simulink model "Control"  (R2024b)
settings: Solver=VariableStepAuto  StartTime=0.0  StopTime=10.0  RelTol=1e-3
values from neighbouring files (symbols this model uses):
  B = [0; 1/m]    [PaT.m]    (also in VanDerPol.m = [0; 1]; phase_portrait_pendulum.m = [0; 1/m*l])
  g = 9.81    [phase_portrait_pendulum.m]
undefined symbols (not defined in the file or in its folder): K, K1, Ke, Kt, L, Lm, m0, m1, N, R, r
settings Model: Creator=Anfisa Konycheva  LastModifiedBy=Anfisa Konycheva

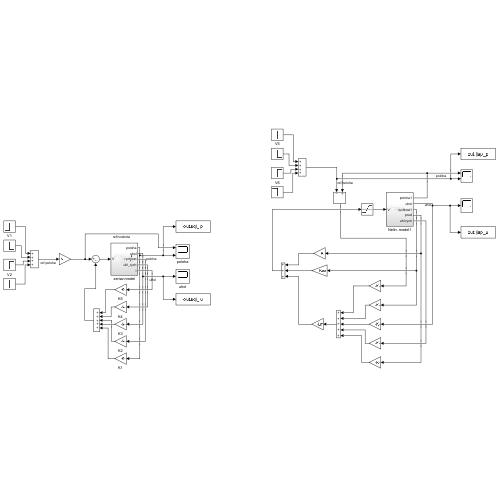
[thumbnail: Simulink's stored preview of the top-level diagram]
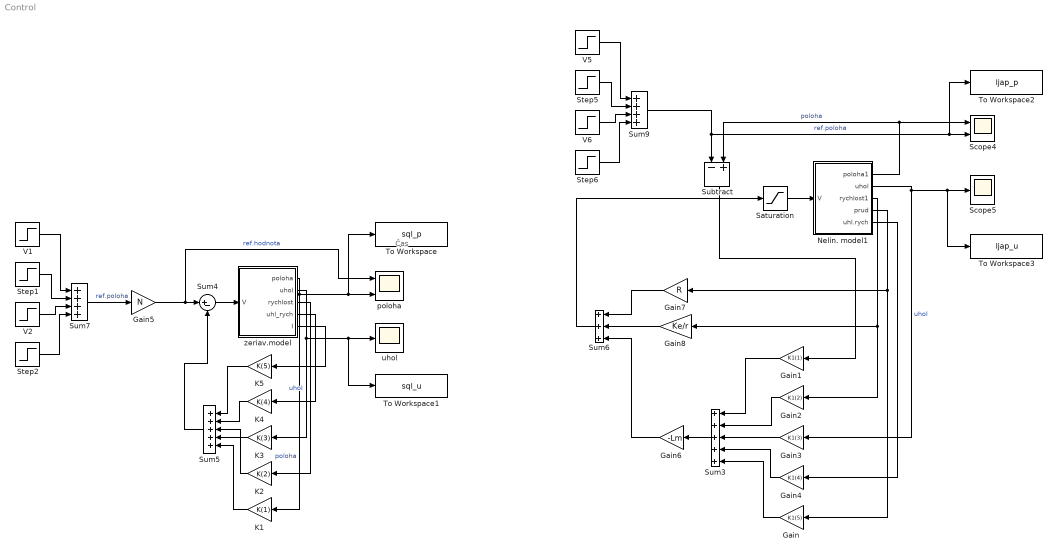
== system Control ==
  note: Čas
  Gain : Gain  Gain=K1(5)
  Gain1 : Gain  Gain=K1(1)
  Gain2 : Gain  Gain=K1(2)
  Gain3 : Gain  Gain=K1(3)
  Gain4 : Gain  Gain=K1(4)
  Gain5 : Gain  Gain=N
  Gain6 : Gain  Gain=-Lm
  Gain7 : Gain  Gain=R
  Gain8 : Gain  Gain=Ke/r
  K1 : Gain  Gain=K(1)
  K2 : Gain  Gain=K(2)
  K3 : Gain  Gain=K(3)
  K4 : Gain  Gain=K(4)
  K5 : Gain  Gain=K(5)
  Nelin. model1 : Subsystem
  Saturation : Saturate  UpperLimit=10  LowerLimit=-10
  Scope4 : Scope  NumInputPorts=2
  Scope5 : Scope
  Step1 : Step  Time=40  After=-5  SampleTime=0
  Step2 : Step  Time=80  After=-5  SampleTime=0
  Step5 : Step  Time=40  After=-5  SampleTime=0
  Step6 : Step  Time=80  After=-5  SampleTime=0
  Subtract : Sum  Inputs=-+
  Sum3 : Sum  Inputs=+++++
  Sum4 : Sum  Inputs=|+-
  Sum5 : Sum  Inputs=+++++
  Sum6 : Sum  Inputs=+++
  Sum7 : Sum  Inputs=++++
  Sum9 : Sum  Inputs=++++
  To Workspace : ToWorkspace  VariableName=sql_p  SaveFormat=Timeseries  SampleTime=-1
  To Workspace1 : ToWorkspace  VariableName=sql_u  SaveFormat=Timeseries  SampleTime=-1
  To Workspace2 : ToWorkspace  VariableName=ljap_p  SaveFormat=Timeseries  SampleTime=-1
  To Workspace3 : ToWorkspace  VariableName=ljap_u  SaveFormat=Timeseries  SampleTime=-1
  V1 : Step  Time=10  After=5  SampleTime=0
  V2 : Step  Time=60  After=5  SampleTime=0
  V5 : Step  Time=10  After=5  SampleTime=0
  V6 : Step  Time=60  After=5  SampleTime=0
  poloha : Scope  NumInputPorts=2
  uhol : Scope
  zeriav.model : Subsystem
  wires:
  K1/1 -> Sum5/5
  zeriav.model/1(poloha) -> K1/1, To Workspace/1, poloha/2  "poloha"
  V5/1 -> Sum9/1
  V6/1 -> Sum9/3
  Saturation/1 -> Nelin. model1/1(V)
  K2/1 -> Sum5/3
  Gain7/1 -> Sum6/1
  K5/1 -> Sum5/1
  Step2/1 -> Sum7/4
  zeriav.model/4(uhl_rych) -> K4/1
  K4/1 -> Sum5/2
  Nelin. model1/3(rychlost1) -> Gain8/1, Gain2/1
  Step5/1 -> Sum9/2
  K3/1 -> Sum5/4
  Step1/1 -> Sum7/2
  Sum6/1 -> Saturation/1
  Sum5/1 -> Sum4/2
  Step6/1 -> Sum9/4
  Gain/1 -> Sum3/5
  zeriav.model/5(I) -> K5/1
  Nelin. model1/1(poloha1) -> Scope4/1, Subtract/2  "poloha"
  Sum7/1 -> Gain5/1  "ref.poloha"
  V2/1 -> Sum7/3
  zeriav.model/3(rychlost) -> K2/1
  Sum3/1 -> Gain6/1
  zeriav.model/2(uhol) -> K3/1, To Workspace1/1, uhol/1  "uhol"
  Gain1/1 -> Sum3/1
  Gain8/1 -> Sum6/2
  Nelin. model1/5(uhl.rych) -> Gain4/1
  Nelin. model1/4(prud) -> Gain7/1, Gain/1
  Sum4/1 -> zeriav.model/1(V)
  Sum9/1 -> Subtract/1, To Workspace2/1, Scope4/2  "ref.poloha"
  Gain4/1 -> Sum3/4
  Gain6/1 -> Sum6/3
  Gain5/1 -> poloha/1, Sum4/1  "ref.hodnota"
  Nelin. model1/2(uhol) -> Gain3/1, To Workspace3/1, Scope5/1  "uhol"
  Gain3/1 -> Sum3/3
  Subtract/1 -> Gain1/1
  Gain2/1 -> Sum3/2
  V1/1 -> Sum7/1

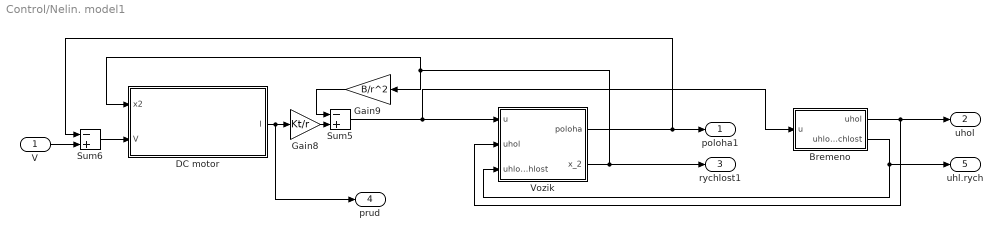
== system Control/Nelin. model1 ==
  V : Inport
  Bremeno : Subsystem
  DC motor : Subsystem
  Gain8 : Gain  Gain=Kt/r
  Gain9 : Gain  Gain=B/r^2
  Sum5 : Sum  Inputs=-+
  Sum6 : Sum  Inputs=-+
  Vozik : Subsystem
  poloha1 : Outport
  uhol : Outport  Port=2
  rychlost1 : Outport  Port=3
  prud : Outport  Port=4
  uhl.rych : Outport  Port=5
  wires:
  V/1 -> Sum6/2
  DC motor/1(I) -> prud/1, Gain8/1
  Gain8/1 -> Sum5/2
  Gain9/1 -> Sum5/1
  Sum6/1 -> DC motor/2(V)
  Bremeno/1(uhol) -> uhol/1, Vozik/2(uhol)
  Bremeno/2(uhlova rychlost) -> uhl.rych/1, Vozik/3(uhlova rychlost)
  Vozik/1(poloha) -> poloha1/1, Sum6/1
  Sum5/1 -> Vozik/1(u), Bremeno/1(u)
  Vozik/2(x_2) -> rychlost1/1, DC motor/1(x2), Gain9/1

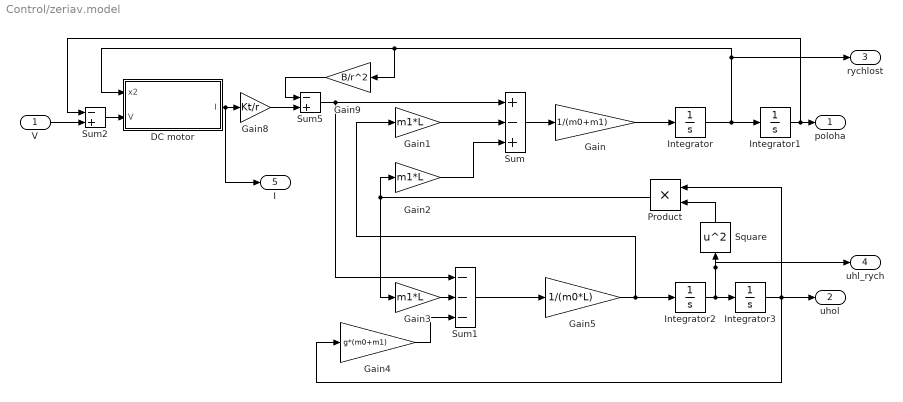
== system Control/zeriav.model ==
  V : Inport
  DC motor : Subsystem
  Gain : Gain  Gain=1/(m0+m1)
  Gain1 : Gain  Gain=m1*L
  Gain2 : Gain  Gain=m1*L
  Gain3 : Gain  Gain=m1*L
  Gain4 : Gain  Gain=g*(m0+m1)
  Gain5 : Gain  Gain=1/(m0*L)
  Gain8 : Gain  Gain=Kt/r
  Gain9 : Gain  Gain=B/r^2
  Integrator{,1..3} (4 alike) : Integrator
  Product : Product
  Square : Math  Operator=square
  Sum : Sum  Inputs=+-+
  Sum1 : Sum  Inputs=---
  Sum2 : Sum  Inputs=-+
  Sum5 : Sum  Inputs=-+
  poloha : Outport
  uhol : Outport  Port=2
  rychlost : Outport  Port=3
  uhl_rych : Outport  Port=4
  I : Outport  Port=5
  wires:
  Square/1 -> Product/2
  Sum5/1 -> Sum1/1, Sum/1
  Gain4/1 -> Sum1/3
  Integrator3/1 -> uhol/1, Gain4/1, Product/1
  Gain3/1 -> Sum1/2
  Integrator/1 -> rychlost/1, DC motor/1(x2), Gain9/1, Integrator1/1
  Product/1 -> Gain2/1, Gain3/1
  Gain1/1 -> Sum/2
  Integrator1/1 -> Sum2/1, poloha/1
  Gain2/1 -> Sum/3
  Gain/1 -> Integrator/1
  Sum/1 -> Gain/1
  Gain5/1 -> Integrator2/1, Gain1/1
  Integrator2/1 -> Integrator3/1, uhl_rych/1, Square/1
  Sum1/1 -> Gain5/1
  V/1 -> Sum2/2
  Gain8/1 -> Sum5/2
  DC motor/1(I) -> I/1, Gain8/1
  Gain9/1 -> Sum5/1
  Sum2/1 -> DC motor/2(V)

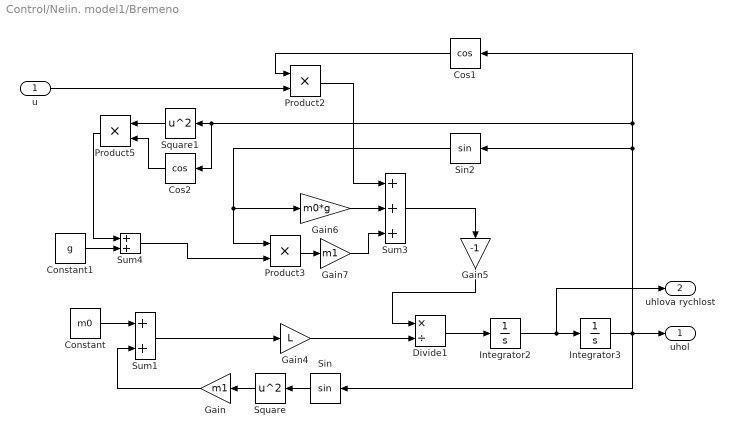
== system Control/Nelin. model1/Bremeno ==
  u : Inport
  Constant : Constant  Value=m0
  Constant1 : Constant  Value=g
  Cos1 : Trigonometry  Operator=cos
  Cos2 : Trigonometry  Operator=cos
  Divide1 : Product  Inputs=*/
  Gain : Gain  Gain=m1
  Gain4 : Gain  Gain=L
  Gain5 : Gain  Gain=-1
  Gain6 : Gain  Gain=m0*g
  Gain7 : Gain  Gain=m1
  Integrator2 : Integrator
  Integrator3 : Integrator
  Product2 : Product
  Product3 : Product
  Product5 : Product
  Sin : Trigonometry
  Sin2 : Trigonometry
  Square : Math  Operator=square
  Square1 : Math  Operator=square
  Sum1 : Sum
  Sum3 : Sum  Inputs=+++
  Sum4 : Sum
  uhol : Outport
  uhlova rychlost : Outport  Port=2
  wires:
  Product5/1 -> Sum4/1
  Gain6/1 -> Sum3/2
  Sum3/1 -> Gain5/1
  Constant1/1 -> Sum4/2
  Sum1/1 -> Gain4/1
  Gain7/1 -> Sum3/3
  Gain5/1 -> Divide1/1
  Product3/1 -> Gain7/1
  Cos2/1 -> Product5/2
  Product2/1 -> Sum3/1
  Sum4/1 -> Product3/2
  Divide1/1 -> Integrator2/1
  Sin2/1 -> Gain6/1, Product3/1
  Gain4/1 -> Divide1/2
  Integrator2/1 -> uhlova rychlost/1, Integrator3/1
  Cos1/1 -> Product2/1
  u/1 -> Product2/2
  Square1/1 -> Product5/1
  Square/1 -> Gain/1
  Constant/1 -> Sum1/1
  Sin/1 -> Square/1
  Gain/1 -> Sum1/2
  Integrator3/1 -> Sin/1, uhol/1, Cos1/1, Cos2/1, Square1/1, Sin2/1

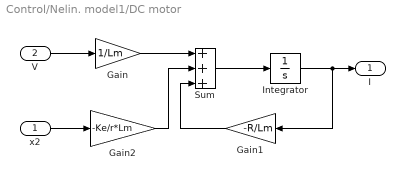
== system Control/Nelin. model1/DC motor ==
  x2 : Inport
  V : Inport  Port=2
  Gain : Gain  Gain=1/Lm
  Gain1 : Gain  Gain=-R/Lm
  Gain2 : Gain  Gain=-Ke/r*Lm
  Integrator : Integrator
  Sum : Sum  Inputs=+++
  I : Outport
  wires:
  V/1 -> Gain/1
  Gain/1 -> Sum/1
  Gain1/1 -> Sum/3
  x2/1 -> Gain2/1
  Gain2/1 -> Sum/2
  Sum/1 -> Integrator/1
  Integrator/1 -> I/1, Gain1/1

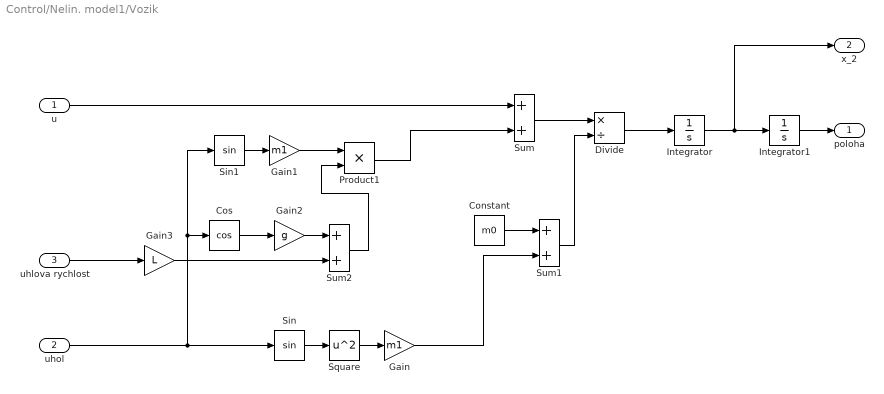
== system Control/Nelin. model1/Vozik ==
  u : Inport
  uhol : Inport  Port=2
  uhlova rychlost : Inport  Port=3
  Constant : Constant  Value=m0
  Cos : Trigonometry  Operator=cos
  Divide : Product  Inputs=*/
  Gain : Gain  Gain=m1
  Gain1 : Gain  Gain=m1
  Gain2 : Gain  Gain=g
  Gain3 : Gain  Gain=L
  Integrator : Integrator
  Integrator1 : Integrator
  Product1 : Product
  Sin : Trigonometry
  Sin1 : Trigonometry
  Square : Math  Operator=square
  Sum : Sum
  Sum1 : Sum
  Sum2 : Sum
  poloha : Outport
  x_2 : Outport  Port=2
  wires:
  Product1/1 -> Sum/2
  Gain1/1 -> Product1/1
  Sin/1 -> Square/1
  Cos/1 -> Gain2/1
  uhol/1 -> Sin/1, Sin1/1, Cos/1
  Integrator/1 -> x_2/1, Integrator1/1
  Sum/1 -> Divide/1
  Divide/1 -> Integrator/1
  Sum1/1 -> Divide/2
  Sum2/1 -> Product1/2
  Gain2/1 -> Sum2/1
  Gain/1 -> Sum1/2
  Constant/1 -> Sum1/1
  Sin1/1 -> Gain1/1
  Gain3/1 -> Sum2/2
  Square/1 -> Gain/1
  Integrator1/1 -> poloha/1
  uhlova rychlost/1 -> Gain3/1
  u/1 -> Sum/1

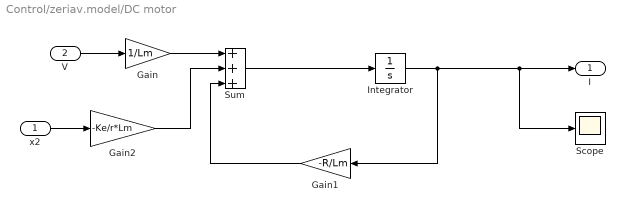
== system Control/zeriav.model/DC motor ==
  x2 : Inport
  V : Inport  Port=2
  Gain : Gain  Gain=1/Lm
  Gain1 : Gain  Gain=-R/Lm
  Gain2 : Gain  Gain=-Ke/r*Lm
  Integrator : Integrator
  Scope : Scope
  Sum : Sum  Inputs=+++
  I : Outport
  wires:
  V/1 -> Gain/1
  Gain/1 -> Sum/1
  Gain1/1 -> Sum/3
  x2/1 -> Gain2/1
  Gain2/1 -> Sum/2
  Sum/1 -> Integrator/1
  Integrator/1 -> Scope/1, I/1, Gain1/1
